simulink library "controlSelection_lib"  (R2018b)
settings: Solver=VariableStepAuto  StartTime=0.0  StopTime=10.0  RelTol=1e-3
libraries: PD_Controller_Lib x2, asmController_lib x1, desat_controller_lib x1, null_control_lib x1, sunSeek_lib x1
settings Model: Creator=Taylor  LastModifiedBy=Nick's PC

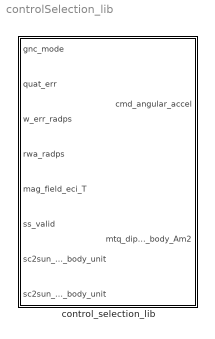
== system controlSelection_lib ==
  control_selection_lib : Subsystem

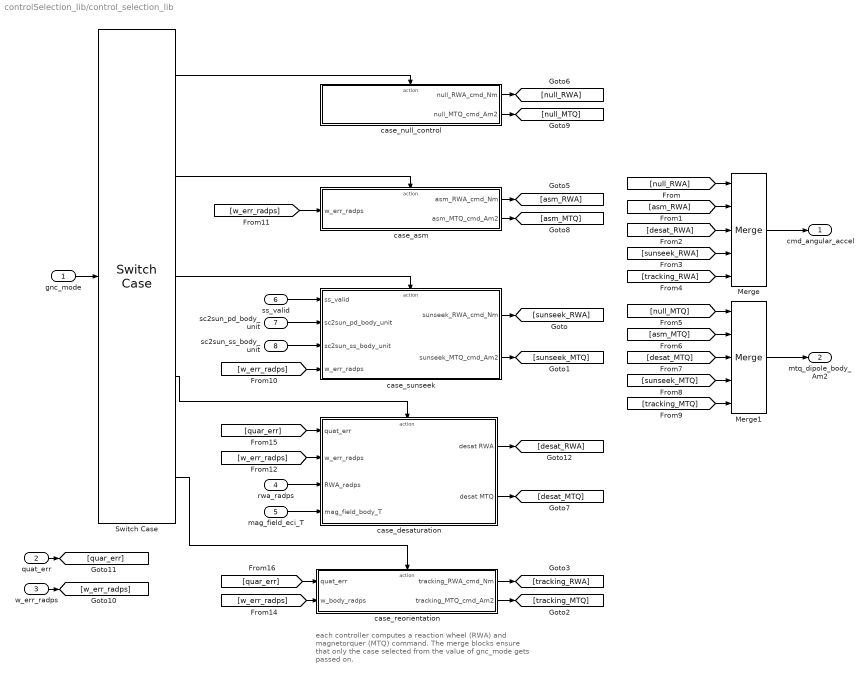
== system controlSelection_lib/control_selection_lib ==
  note: each controller computes a reaction wheel (RWA) and
      | magnetorquer (MTQ) command. The merge blocks
      | ensure that only the case selected from the value of
      | gnc_mode gets passed on.
  gnc_mode : Inport
  quat_err : Inport  Port=2
  w_err_radps : Inport  Port=3
  rwa_radps : Inport  Port=4
  mag_field_eci_T : Inport  Port=5
  ss_valid : Inport  Port=6
  sc2sun_pd_body_unit : Inport  Port=7
  sc2sun_ss_body_unit : Inport  Port=8
  Merge : Merge  Inputs=5
  Merge1 : Merge  Inputs=5
  Switch Case : SwitchCase  CaseConditions={[0,1,2,4],3,5,[6],[7,8]}  ShowDefaultCase=off  ZeroCross=off
  case_asm : Subsystem  TreatAsAtomicUnit=on
  case_desaturation : Subsystem  TreatAsAtomicUnit=on
  case_null_control : Subsystem  TreatAsAtomicUnit=on
  case_reorientation : Subsystem  TreatAsAtomicUnit=on
  case_sunseek : Subsystem  TreatAsAtomicUnit=on
  cmd_angular_accel : Outport
  mtq_dipole_body_Am2 : Outport  Port=2
  wires:
  gnc_mode/1 -> Switch Case/1
  mag_field_eci_T/1 -> case_desaturation/4(mag_field_body_T)
  Switch Case/2 -> case_asm/Action
  rwa_radps/1 -> case_desaturation/3(RWA_radps)
  Switch Case/1 -> case_null_control/Action
  Merge1/1 -> mtq_dipole_body_Am2/1
  Merge/1 -> cmd_angular_accel/1
  case_sunseek/1(sunseek_RWA_cmd_Nm) -> [sunseek_RWA]
  case_sunseek/2(sunseek_MTQ_cmd_Am2) -> [sunseek_MTQ]
  sc2sun_ss_body_unit/1 -> case_sunseek/3(sc2sun_ss_body_unit)
  ss_valid/1 -> case_sunseek/1(ss_valid)
  sc2sun_pd_body_unit/1 -> case_sunseek/2(sc2sun_pd_body_unit)
  case_asm/1(asm_RWA_cmd_Nm) -> [asm_RWA]
  case_null_control/1(null_RWA_cmd_Nm) -> [null_RWA]
  case_desaturation/2(desat MTQ) -> [desat_MTQ]
  case_asm/2(asm_MTQ_cmd_Am2) -> [asm_MTQ]
  case_null_control/2(null_MTQ_cmd_Am2) -> [null_MTQ]
  [null_RWA] -> Merge/1
  [asm_RWA] -> Merge/2
  [desat_RWA] -> Merge/3
  [sunseek_RWA] -> Merge/4
  [tracking_RWA] -> Merge/5
  [null_MTQ] -> Merge1/1
  [asm_MTQ] -> Merge1/2
  [desat_MTQ] -> Merge1/3
  [sunseek_MTQ] -> Merge1/4
  [tracking_MTQ] -> Merge1/5
  Switch Case/5 -> case_reorientation/Action
  case_reorientation/1(tracking_RWA_cmd_Nm) -> [tracking_RWA]
  case_reorientation/2(tracking_MTQ_cmd_Am2) -> [tracking_MTQ]
  Switch Case/3 -> case_sunseek/Action
  Switch Case/4 -> case_desaturation/Action
  w_err_radps/1 -> [w_err_radps]
  [w_err_radps] -> case_asm/1(w_err_radps)
  [w_err_radps] -> case_desaturation/2(w_err_radps)
  [w_err_radps] -> case_reorientation/2(w_body_radps)
  quat_err/1 -> [quar_err]
  [quar_err] -> case_desaturation/1("quat_err ")
  [quar_err] -> case_reorientation/1(quat_err)
  case_desaturation/1(desat RWA) -> [desat_RWA]
  [w_err_radps] -> case_sunseek/4(w_err_radps)

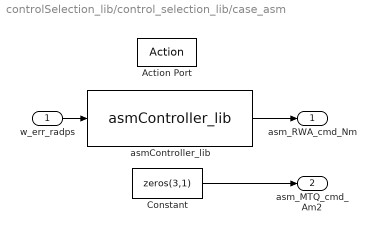
== system controlSelection_lib/control_selection_lib/case_asm ==
  w_err_radps : Inport
  Action Port : ActionPort  ActionType=case
  Constant : Constant  Value=zeros(3,1)
  asmController_lib : asmController_lib/asmController_lib  SystemSampleTime=-1
  asm_RWA_cmd_Nm : Outport
  asm_MTQ_cmd_Am2 : Outport  Port=2
  wires:
  w_err_radps/1 -> asmController_lib/1
  asmController_lib/1 -> asm_RWA_cmd_Nm/1
  Constant/1 -> asm_MTQ_cmd_Am2/1

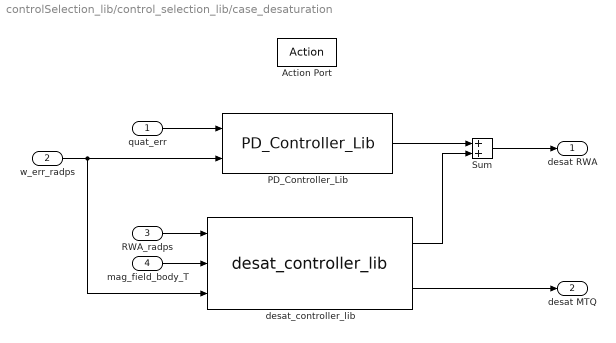
== system controlSelection_lib/control_selection_lib/case_desaturation ==
  "quat_err " : Inport
  w_err_radps : Inport  Port=2
  RWA_radps : Inport  Port=3
  mag_field_body_T : Inport  Port=4
  Action Port : ActionPort  ActionType=case
  PD_Controller_Lib : PD_Controller_Lib/PD_Controller_Lib  SystemSampleTime=-1
  Sum : Sum
  desat_controller_lib : desat_controller_lib/desat_controller_lib  SystemSampleTime=-1
  desat RWA : Outport
  desat MTQ : Outport  Port=2
  wires:
  "quat_err "/1 -> PD_Controller_Lib/1
  w_err_radps/1 -> desat_controller_lib/3, PD_Controller_Lib/2
  RWA_radps/1 -> desat_controller_lib/1
  mag_field_body_T/1 -> desat_controller_lib/2
  PD_Controller_Lib/1 -> Sum/1
  desat_controller_lib/1 -> Sum/2
  Sum/1 -> desat RWA/1
  desat_controller_lib/2 -> desat MTQ/1

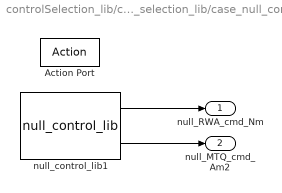
== system controlSelection_lib/control_selection_lib/case_null_control ==
  Action Port : ActionPort  ActionType=case
  null_control_lib1 : null_control_lib/null_control_lib  SystemSampleTime=-1
  null_RWA_cmd_Nm : Outport
  null_MTQ_cmd_Am2 : Outport  Port=2
  wires:
  null_control_lib1/1 -> null_RWA_cmd_Nm/1
  null_control_lib1/2 -> null_MTQ_cmd_Am2/1

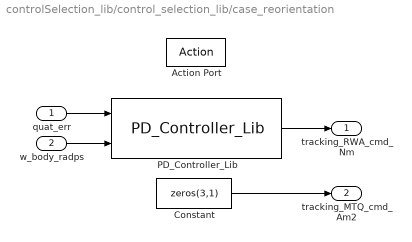
== system controlSelection_lib/control_selection_lib/case_reorientation ==
  quat_err : Inport
  w_body_radps : Inport  Port=2
  Action Port : ActionPort  ActionType=case
  Constant : Constant  Value=zeros(3,1)
  PD_Controller_Lib : PD_Controller_Lib/PD_Controller_Lib  SystemSampleTime=-1
  tracking_RWA_cmd_Nm : Outport
  tracking_MTQ_cmd_Am2 : Outport  Port=2
  wires:
  PD_Controller_Lib/1 -> tracking_RWA_cmd_Nm/1
  quat_err/1 -> PD_Controller_Lib/1
  w_body_radps/1 -> PD_Controller_Lib/2
  Constant/1 -> tracking_MTQ_cmd_Am2/1

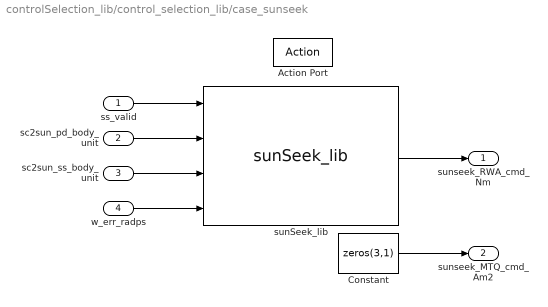
== system controlSelection_lib/control_selection_lib/case_sunseek ==
  ss_valid : Inport
  sc2sun_pd_body_unit : Inport  Port=2
  sc2sun_ss_body_unit : Inport  Port=3
  w_err_radps : Inport  Port=4
  Action Port : ActionPort  ActionType=case
  Constant : Constant  Value=zeros(3,1)
  sunSeek_lib : sunSeek_lib/sunSeek_lib  SystemSampleTime=-1
  sunseek_RWA_cmd_Nm : Outport
  sunseek_MTQ_cmd_Am2 : Outport  Port=2
  wires:
  sunSeek_lib/1 -> sunseek_RWA_cmd_Nm/1
  Constant/1 -> sunseek_MTQ_cmd_Am2/1
  ss_valid/1 -> sunSeek_lib/1
  w_err_radps/1 -> sunSeek_lib/4
  sc2sun_ss_body_unit/1 -> sunSeek_lib/3
  sc2sun_pd_body_unit/1 -> sunSeek_lib/2
